simulink model "Approx_Adder_Template_1"  (R2021a)
settings: Solver=VariableStepAuto  StartTime=0.0  StopTime=10.0  RelTol=1e-3
settings Model: Creator=mohandassakthi  LastModifiedBy=mohandassakthi

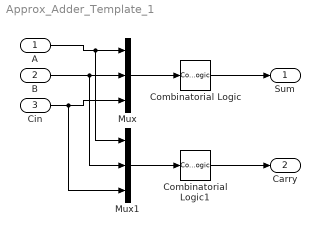
== system Approx_Adder_Template_1 ==
  A : Inport
  B : Inport  Port=2
  Cin : Inport  Port=3
  Combinatorial Logic : CombinatorialLogic
  Combinatorial Logic1 : CombinatorialLogic
  Mux : Mux  Inputs=3
  Mux1 : Mux  Inputs=3
  Sum : Outport
  Carry : Outport  Port=2
  wires:
  A/1 -> Mux1/1, Mux/1
  B/1 -> Mux1/2, Mux/2
  Cin/1 -> Mux1/3, Mux/3
  Mux/1 -> Combinatorial Logic/1
  Mux1/1 -> Combinatorial Logic1/1
  Combinatorial Logic/1 -> Sum/1
  Combinatorial Logic1/1 -> Carry/1
